simulink model "Solar_Tracker_ProjectV3"  (R2025a)
settings: Solver=ode23tb  StartTime=0.0  StopTime=1  FixedStep=1e-8  MaxStep=1e-6  RelTol=1e-3
libraries: spsSeriesRLCBranchLib x4, spsCurrentMeasurementLib x2, spsVoltageMeasurementLib x2, spsDCVoltageSourceLib x1, spsDiodeLib x1, spsIGBTLib x1, slpidlib x1, spsPVArrayLib x1, spsPWMGeneratorDCDCLib x1, spspowerguiLib x1
settings Model: Creator=fahad  LastModifiedBy=fahad

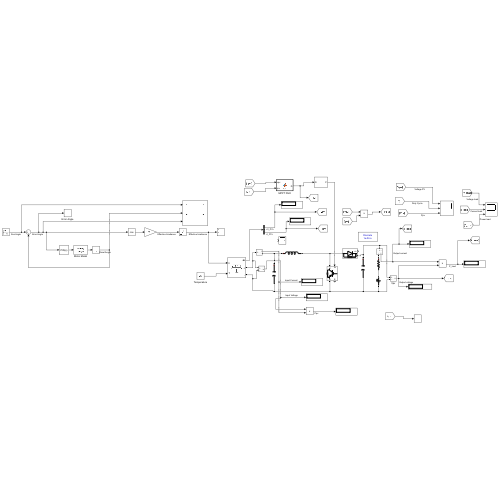
[thumbnail: Simulink's stored preview of the top-level diagram]
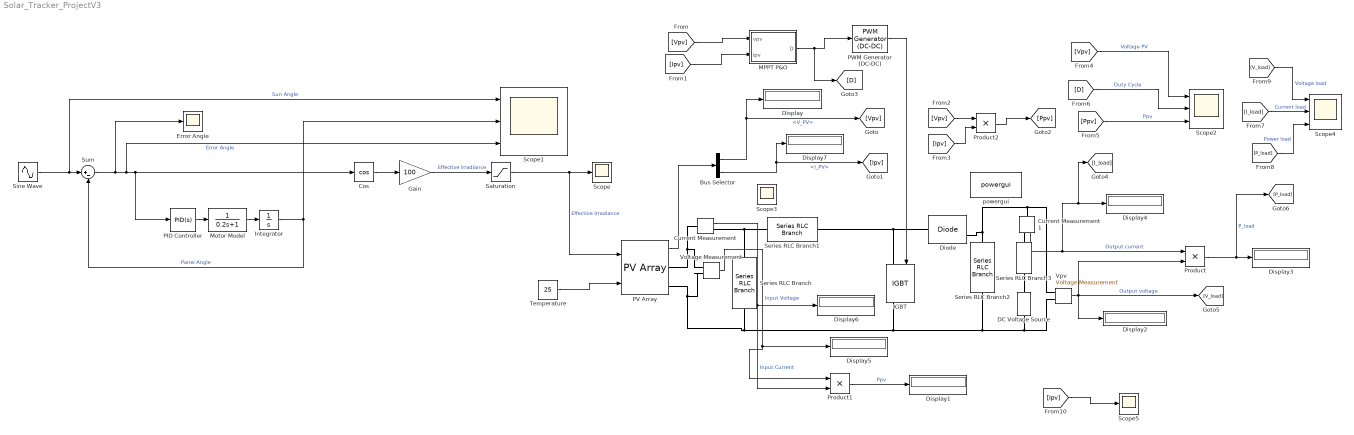
== system Solar_Tracker_ProjectV3 ==
  Bus Selector : BusSelector  OutputSignals=V_PV,I_PV
  Cos : Trigonometry  Operator=cos
  Current Measurement : spsCurrentMeasurementLib/Current Measurement  PhasorSimulation=off  OutputType=Complex  PSBequivalent=0
  Current Measurement1 : spsCurrentMeasurementLib/Current Measurement  PhasorSimulation=off  OutputType=Complex  PSBequivalent=0
  DC Voltage Source : spsDCVoltageSourceLib/DC Voltage Source  Amplitude=48  Measurements=None
  Diode : spsDiodeLib/Diode  Ron=0.001  Lon=0  Vf=0.8  IC=0  UseSnubber=0  Rs=500  Cs=250e-9  Measurements=on
  Display{,1..7} (8 alike) : Display
  Error Angle : Scope
      settings: ActiveDisplayYMinimum=-1  ActiveDisplayYMaximum=1  DataLoggingVariableName=ScopeData2
  Gain : Gain  Gain=100
  IGBT : spsIGBTLib/IGBT  Ron=0.001  Lon=0  Vf=1  Tf=1e-6  Tt=2e-6  IC=0  Rs=1e5  Cs=inf  Measurements=on
  Integrator : Integrator
  MPPT P&O : MATLAB Function  TreatAsAtomicUnit=on
  Motor Model : TransferFcn  Denominator=[0.2 1]
  PID Controller : slpidlib/PID Controller  Controller=PID  Form=Parallel  TimeDomain=Continuous-time  UseExternalTs=off  SampleTime=-1  IntegratorMethod=Forward Euler  FilterMethod=Forward Euler  ControllerParametersSource=internal  P=100  I=70  UseKiTs=off  D=0  UseExternalDerivativeSource=off  N=100  UseFilter=on  TunerSelectOption=Transfer Function Based (PID Tuner App)  InitialConditionSource=internal  InitialConditionForIntegrator=0  InitialConditionForFilter=0  DifferentiatorICPrevScaledInput=0  ExternalReset=none  TrackingMode=off  Kt=1  LimitOutput=off  SatLimitsSource=internal  UpperSaturationLimit=inf  LowerSaturationLimit=-inf  LinearizeAsGain=on  AntiWindupMode=none  Kb=1  LimitIntegrator=off  UpperIntegratorSaturationLimit=inf  LowerIntegratorSaturationLimit=-inf  POutMin=[]  POutMax=[]  IOutMin=[]  IOutMax=[]  DOutMin=[]  DOutMax=[]  NOutMin=[]  NOutMax=[]  SumOutMin=[]  SumOutMax=[]  SaturationOutMin=[]  SaturationOutMax=[]  PParamMin=[]  PParamMax=[]  IParamMin=[]  IParamMax=[]  DParamMin=[]  DParamMax=[]  NParamMin=[]  NParamMax=[]  KbParamMin=[]  KbParamMax=[]  KtParamMin=[]  KtParamMax=[]  KbOutMin=[]  KbOutMax=[]  KtOutMin=[]  KtOutMax=[]  IntegratorOutMin=[]  IntegratorOutMax=[]  FilterOutMin=[]  FilterOutMax=[]  SumI1OutMin=[]  SumI1OutMax=[]  SumI2OutMin=[]  SumI2OutMax=[]  SumI3OutMin=[]  SumI3OutMax=[]  SumI4OutMin=[]  SumI4OutMax=[]  SumDOutMin=[]  SumDOutMax=[]  DifferentiatorOutMin=[]  DifferentiatorOutMax=[]  FilterDiffOutCoefMin=[]  FilterDiffOutCoefMax=[]  ReciprocalOutMin=[]  ReciprocalOutMax=[]  SumDenOutMin=[]  SumDenOutMax=[]  SumNumOutMin=[]  SumNumOutMax=[]  DivideOutMin=[]  DivideOutMax=[]  UdiffTsProdOutMin=[]  UdiffTsProdOutMax=[]  NTsProdOutMin=[]  NTsProdOutMax=[]  UintegralTsProdOutMin=[]  UintegralTsProdOutMax=[]  UngainTsProdOutMin=[]  UngainTsProdOutMax=[]  ClampingZeroOutDataTypeStr=Inherit: Inherit via back propagation  ClampingZeroOutMin=[]  ClampingZeroOutMax=[]  FilterDenConstantOutDataTypeStr=Inherit: Inherit via back propagation  FilterDenConstantOutMin=[]  FilterDenConstantOutMax=[]  PCopyOutDataTypeStr=Inherit: Inherit via back propagation  PCopyOutMin=[]  PCopyOutMax=[]  NCopyOutDataTypeStr=Inherit: Inherit via back propagation  NCopyOutMin=[]  NCopyOutMax=[]  IntegratorContinuousStateAttributes=''  IntegratorStateMustResolveToSignalObject=off  IntegratorRTWStateStorageClass=Auto  FilterContinuousStateAttributes=''  FilterStateMustResolveToSignalObject=off  FilterRTWStateStorageClass=Auto  ParallelPVariant=InternalParameters  IdealPVariant=Disabled  IVariant=InternalParameters  DVariant=InternalParameters  IntegratorVariant=Continuous  SatVariant=Disabled  AWVariant=Passthrough  PCopyVariant=Disabled  TRVariant=Disabled  FdbkBlocksVariant=Forward  IdealPFdbkVariant=Disabled  SatFdbkVariant=Disabled  DerivativeFilterVariant=ContFilter  NVariant=InternalParameters  NCopyVariant=Disabled  FilterICVariant=InternalICsFilter  IntegratorICVariant=InternalICs  ExternalResetVariant=Disabled  TRSumVariant=Passthrough  SumFdbkVariant=Disabled  SumVariant=Sum_PID  TsampFilterVariant=InternalTs  TsampNgainVariant=Passthrough  TsampIntegralVariant=Disabled_SignalSpec  ExternalSaturationOutDataTypeStr=Inherit: Same as second input  DerivativeSourceVariant=ErrorSignal  PreIntVariant=InternalPreInt
  PV Array : spsPVArrayLib/PV Array  Npar=1  Nser=1  PlotType=array @ 25 deg.C & specified irradiances  S_vec="[ 1000  500  100 ]"  Temp_C_vec="[ 45 25  ]"  ModuleName=User-defined  PlotWhenSelected=off  Pm=213.15  Ncell=60  Voc=36.3  Isc=7.84  Vm=29  Im=7.35  beta_Voc_pc=-0.36099  alpha_Isc_pc=0.102  beta_Voc=-0.13104  alpha_Isc=0.0079968  IL=7.8654  I0=2.9273e-10  nI=0.98119  Rsh=313.0553  Rs=0.39381  RobustModel=off  RobustCellTemperature=313.3991  BAL=on  Tc=1e-6  Tfilter=5e-5
  PWM Generator (DC-DC) : spsPWMGeneratorDCDCLib/PWM Generator (DC-DC)  Fsw=5000  Ts=1e-5
  Product : Product
  Product1 : Product
  Product2 : Product
  Saturation : Saturate  UpperLimit=1000  LowerLimit=0
  Scope : Scope
      settings: ActiveDisplayYMinimum=99.877948156214  ActiveDisplayYMaximum=100.01356131597623
  Scope1 : Scope  NumInputPorts=3
      settings: ActiveDisplayYMinimum=-0.12945365000660086  ActiveDisplayYMaximum=0.94994059023460875
  Scope2 : Scope  NumInputPorts=3
      settings: ActiveDisplayYMinimum=-4.0226761621871052  ActiveDisplayYMaximum=36.2434099361278  DataLoggingVariableName=ScopeData3
  Scope3 : Scope
      settings: ActiveDisplayYMinimum=-0.027349487232342984  ActiveDisplayYMaximum=1.0103527854363679  DataLoggingVariableName=ScopeData4
  Scope4 : Scope  NumInputPorts=3
      settings: ActiveDisplayYMinimum=47.5829793737067  ActiveDisplayYMaximum=51.753185636950349  DataLoggingVariableName=ScopeData5
  Scope5 : Scope
      settings: ActiveDisplayYMinimum=-14.898179945206305  ActiveDisplayYMaximum=10.394067233569052  DataLoggingVariableName=ScopeData6
  Series RLC Branch : spsSeriesRLCBranchLib/Series RLC Branch  LConnTagsString=__new0  RConnTagsString=__new0  BranchType=C  Resistance=1  Inductance=1e-3  SetiL0=off  InitialCurrent=0  Capacitance=100e-6  Setx0=off  InitialVoltage=0  Measurements=None
  Series RLC Branch1 : spsSeriesRLCBranchLib/Series RLC Branch  LConnTagsString=__new0  RConnTagsString=__new0  BranchType=L  Resistance=1  Inductance=5e-3  SetiL0=off  InitialCurrent=0  Capacitance=100e-6  Setx0=off  InitialVoltage=0  Measurements=None
  Series RLC Branch2 : spsSeriesRLCBranchLib/Series RLC Branch  LConnTagsString=__new0  RConnTagsString=__new0  BranchType=C  Resistance=1  Inductance=1e-3  SetiL0=off  InitialCurrent=0  Capacitance=6000e-6  Setx0=off  InitialVoltage=0  Measurements=None
  Series RLC Branch3 : spsSeriesRLCBranchLib/Series RLC Branch  LConnTagsString=__new0  RConnTagsString=__new0  BranchType=R  Resistance=10  Inductance=1e-3  SetiL0=off  InitialCurrent=0  Capacitance=220e-6  Setx0=off  InitialVoltage=0  Measurements=None
  Sine Wave : Sin  SampleTime=0
  Sum : Sum  Inputs=|+-
  Temperature : Constant  Value=25
  Voltage Measurement : spsVoltageMeasurementLib/Voltage Measurement  PhasorSimulation=off  OutputType=Complex  PSBequivalent=0
  Vpv : spsVoltageMeasurementLib/Voltage Measurement  PhasorSimulation=off  OutputType=Complex  PSBequivalent=0
  powergui : spspowerguiLib/powergui  Priority=1  SimulationMode=Discrete  SampleTime=1e-6  frequency=60  Iterations=50  frequencyindice=0  Pbase=100e6  ErrMax=1e-4  UnitsV=kV  UnitsW=MW  buscounter=0  FunctionMessages=off  echomessages=off  EnableUseOfTLC=off  CurrentSourceSwitches=off  DisableSnubberDevices=off  DisableRonSwitches=off  DisableVfSwitches=off  DisplayEquations=off  AutomaticDiscreteSolvers=off  SolverType=Tustin/Backward Euler (TBE)  Interpol=off  ExternalGateDelay=off  methode=off  Ts=100  x0status=blocks  SPID=on  SwTol=0  HookPort=off  NonlinearTolerance=1e-4  nMaxIteration=100  ContinueOnMaxIteration=off  RestoreLinks=warning  ResistiveCurrentMeasurement=off  Frange=[0:2:500]  Ylog=off  Xlog=on  ShowGrid=off  save=off  variable=ZData  structure=0  ZoomFFT=off  StartTime=0.0  cycles=1  DisplayStyle=1  fundamental=60  FreqAxis=off  MaxFrequency=1000  frequencyindicesteady=1  RmsSteady=1  display=off
  wires:
  Sine Wave/1 -> Scope1/1, Sum/1  "Sun Angle"
  Sum/1 -> Cos/1, PID Controller/1, Scope1/3, Error Angle/1  "Error Angle"
  Gain/1 -> Saturation/1  "Effective Irradiance"
  Saturation/1 -> PV Array/1, Scope/1  "Effective Irradiance"
  Cos/1 -> Gain/1
  Integrator/1 -> Sum/2, Scope1/2  "Panel Angle"
  PID Controller/1 -> Motor Model/1
  Motor Model/1 -> Integrator/1
  Temperature/1 -> PV Array/2
  Vpv/1 -> Product/2, [V_load], Display2/1  "Output voltage"
  Product/1 -> [P_load], Display3/1  "P_load"
  Voltage Measurement/1 -> Product1/1, Display5/1  "Input Voltage"
  Current Measurement1/1 -> Product/1, [I_load], Display4/1  "Output current"
  Current Measurement/1 -> Product1/2, Display6/1  "Input Current"
  Product1/1 -> Display1/1  "Ppv"
  PV Array/1 -> Bus Selector/1
  Bus Selector/1 -> [Vpv], Display/1  "<V_PV>"
  Bus Selector/2 -> [Ipv], Display7/1  "<I_PV>"
  PWM Generator (DC-DC)/1 -> IGBT/1
  Product2/1 -> [Ppv]
  [Vpv] -> Product2/1
  [Ipv] -> Product2/2
  [Vpv] -> Scope2/1  "Voltage PV"
  [Ppv] -> Scope2/3  "Ppv"
  [D] -> Scope2/2  "Duty Cycle"
  [I_load] -> Scope4/2  "Current load"
  [P_load] -> Scope4/3  "Power load"
  [V_load] -> Scope4/1  "Voltage load"
  [Ipv] -> Scope5/1
  MPPT P&O/1(D) -> [D], PWM Generator (DC-DC)/1
  [Vpv] -> MPPT P&O/1(vpv)
  [Ipv] -> MPPT P&O/2(ipv)
  connections:
  Diode/LConn1 -- IGBT/LConn1 -- Series RLC Branch1/RConn1
  Vpv/LConn1 -- Current Measurement1/LConn1 -- Diode/RConn1 -- Series RLC Branch2/LConn1
  IGBT/RConn1 -- Series RLC Branch/RConn1 -- PV Array/RConn2 -- Voltage Measurement/LConn2 -- Series RLC Branch2/RConn1 -- DC Voltage Source/LConn1 -- Vpv/LConn2
  Series RLC Branch3/LConn1 -- Current Measurement1/RConn1
  Voltage Measurement/LConn1 -- Current Measurement/LConn1 -- PV Array/RConn1
  Current Measurement/RConn1 -- Series RLC Branch/LConn1 -- Series RLC Branch1/LConn1
  Series RLC Branch3/RConn1 -- DC Voltage Source/RConn1

== matlab function Solar_Tracker_ProjectV3/MPPT P&O ==
  data: vpv input; D output; ipv input
function D = fcn(vpv,ipv)
Dinit = 0.4;
Dmax = 0.9;
Dmin = 0.1;
deltaD = 20e-6;

persistent Vold Pold Dold;
dataType = "double";
if isempty(Vold)
    Vold = 0;
    Pold = 0;
    Dold = Dinit;
end
P = vpv*ipv;
dV = vpv-Vold;
dP= P-Pold;
if dP ~= 0
    if dP < 0
        if dV < 0
            D = Dold-deltaD;
        else
            D = Dold + deltaD;
        end
        else
        if dV < 0
            D = Dold + deltaD;
        else
            D = Dold - deltaD;
        end
    end
else 
    D = Dold;
end
if D >= Dmax || D <= Dmin
    D = Dold;
end

Dold=D;
Vold=vpv;
Pold=P;
